simulink subsystem "MotorCtrl"  (R2023b)
settings: Solver=VariableStepAuto  StartTime=0.0  StopTime=10.0  RelTol=1e-3
libraries: simulink x2
settings Model: Creator=m4ttn  LastModifiedBy=m4ttn
settings RTWCC: GPUComputeCapability=5.0

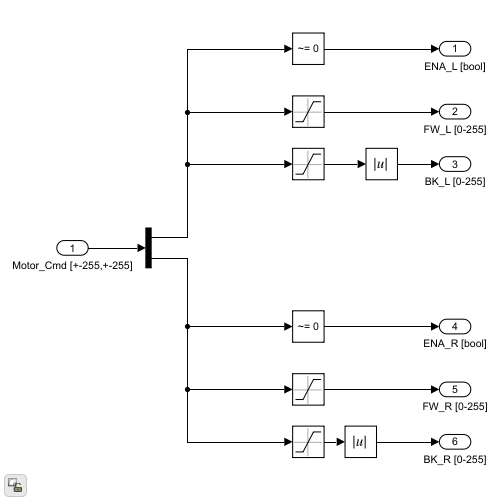
[thumbnail: Simulink's stored preview of the top-level diagram]
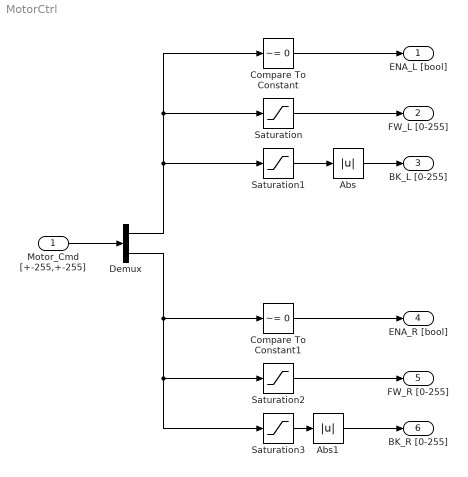
== system MotorCtrl ==
  Motor_Cmd [+-255,+-255] : Inport  OutDataTypeStr=int16
  Abs : Abs  OutDataTypeStr=uint8  SaturateOnIntegerOverflow=off
  Abs1 : Abs  OutDataTypeStr=uint8  SaturateOnIntegerOverflow=off
  Compare To Constant : simulink/Logic and Bit Operations/Compare To Constant  relop=~=  const=0  OutDataTypeStr=uint8
  Compare To Constant1 : simulink/Logic and Bit Operations/Compare To Constant  relop=~=  const=0  OutDataTypeStr=uint8
  Demux : Demux  Outputs=2
  Saturation : Saturate  UpperLimit=255  LowerLimit=0  OutDataTypeStr=uint8
  Saturation1 : Saturate  UpperLimit=0  LowerLimit=-255  OutDataTypeStr=int16
  Saturation2 : Saturate  UpperLimit=255  LowerLimit=0  OutDataTypeStr=uint8
  Saturation3 : Saturate  UpperLimit=0  LowerLimit=-255  OutDataTypeStr=int16
  ENA_L [bool] : Outport  OutDataTypeStr=uint8
  FW_L [0-255] : Outport  Port=2  OutDataTypeStr=uint8
  BK_L [0-255] : Outport  Port=3  OutDataTypeStr=uint8
  ENA_R [bool] : Outport  Port=4  OutDataTypeStr=uint8
  FW_R [0-255] : Outport  Port=5  OutDataTypeStr=uint8
  BK_R [0-255] : Outport  Port=6  OutDataTypeStr=uint8
  wires:
  Motor_Cmd [+-255,+-255]/1 -> Demux/1
  Saturation/1 -> FW_L [0-255]/1
  Compare To Constant/1 -> ENA_L [bool]/1
  Saturation1/1 -> Abs/1
  Demux/1 -> Saturation1/1, Compare To Constant/1, Saturation/1
  Saturation3/1 -> Abs1/1
  Compare To Constant1/1 -> ENA_R [bool]/1
  Saturation2/1 -> FW_R [0-255]/1
  Demux/2 -> Saturation3/1, Saturation2/1, Compare To Constant1/1
  Abs/1 -> BK_L [0-255]/1
  Abs1/1 -> BK_R [0-255]/1
